simulink model "throttle"  (R2023a)
settings: Solver=VariableStepAuto  StartTime=0.0  StopTime=20.0  RelTol=1e-3
model workspace (MAT data in the model file):
  J = 0.000245
settings Model: Creator=Administrator  LastModifiedBy=Administrator
settings DataIOCC: ExternalInput=[t, direction, duty]  LoadExternalInput=on  SaveState=on

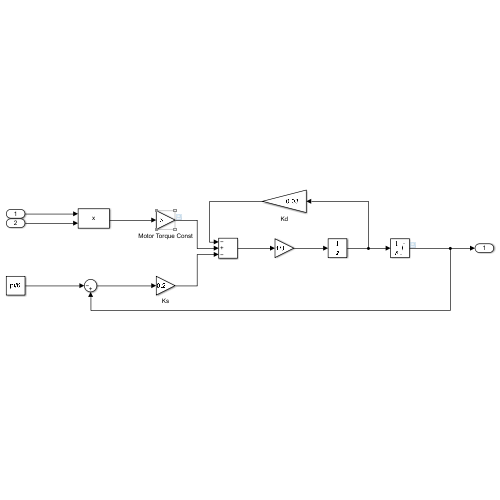
[thumbnail: Simulink's stored preview of the top-level diagram]
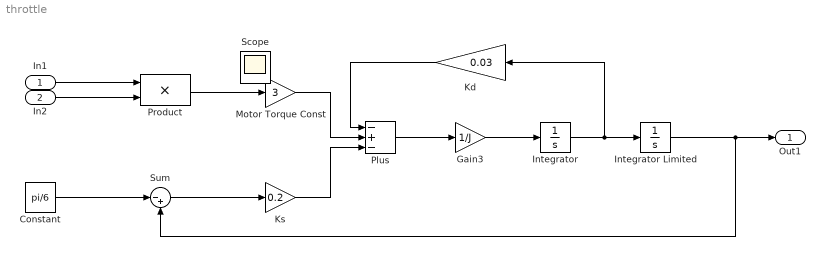
== system throttle ==
  In1 : Inport
  In2 : Inport  Port=2
  Constant : Constant  Value=pi/6
  Gain3 : Gain  Gain=1/J
  Integrator : Integrator
  Integrator Limited : Integrator  InitialCondition=pi/6  LimitOutput=on  UpperSaturationLimit=pi/2  LowerSaturationLimit=0
  Kd : Gain  Gain=0.03
  Ks : Gain  Gain=0.2
  Motor Torque Const : Gain  Gain=3
  Plus : Sum  Inputs=-+-
  Product : Product
  Sum : Sum  Inputs=|-+
  Out1 : Outport
  Scope : Scope
  wires:
  In1/1 -> Product/1
  In2/1 -> Product/2
  Product/1 -> Motor Torque Const/1
  Constant/1 -> Sum/1
  Sum/1 -> Ks/1
  Ks/1 -> Plus/3
  Motor Torque Const/1 -> Plus/2
  Kd/1 -> Plus/1
  Plus/1 -> Gain3/1
  Gain3/1 -> Integrator/1
  Integrator/1 -> Kd/1, Integrator Limited/1
  Integrator Limited/1 -> Sum/2, Out1/1
